simulink model "satPropWThrusterControlLinear"  (R2015b)
settings: Solver=ode45  StartTime=0.0  StopTime=tprop  RelTol=1e-8  AbsTol=1e-8
values from neighbouring files (symbols this model uses):
  epsilon0 = q(2:4)    [SetUp.m]
  eta0 = q(1)    [SetUp.m]
  J = [3500 0 0; 0 3200 0; 0 0 2500]    [SetUp.m]
  Jinv = inv(J)    [SetUp.m]
  kd = J*2*zeta*nf    [SetUp.m]
  kp = J*2*nf^2    [SetUp.m]
  mu = 398600    [COES2rvd.m]    (also in SetUp.m; test.m)
  n = 1/T    [SetUp.m]
  rvect = invconvmat*rvectx    [COES2rvd.m]    (also in test.m = rvect')
  vvect = invconvmat*vvectx    [COES2rvd.m]    (also in test.m = vvect')
  wbn0 = DCM*w    [SetUp.m]
settings Model: Creator=morganyost  LastModifiedBy=morganyost

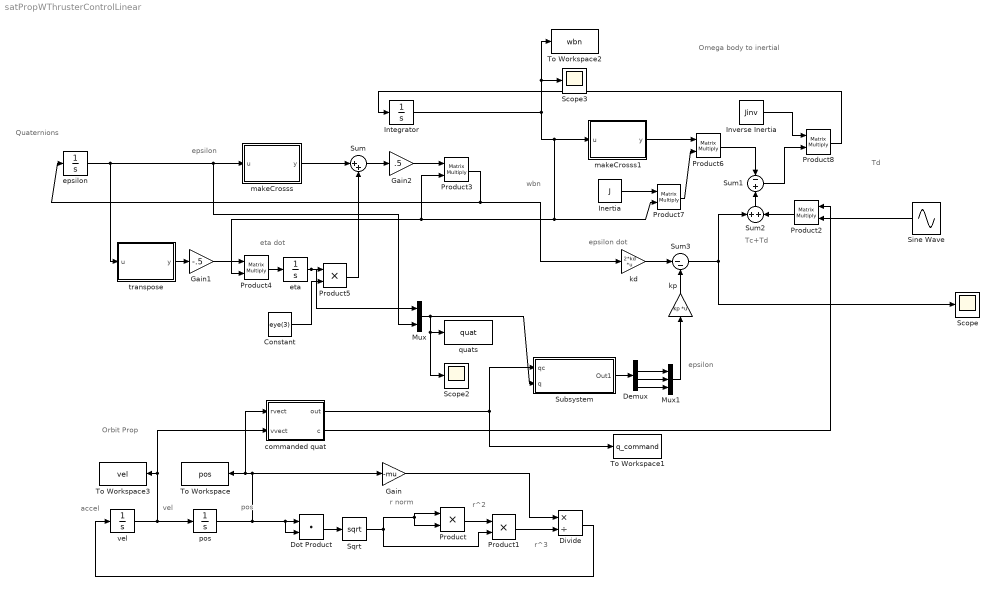
== system satPropWThrusterControlLinear ==
  note: epsilon
  note: epsilon dot
  note: Td
  note: Tc+Td
  note: Quaternions
  note: Omega body to inertial
  note: Orbit Prop
  note: eta dot
  note: wbn
  note: epsilon
  note: r^3
  note: r^2
  note: r norm
  note: pos
  note: vel
  note: accel
  Constant : Constant  Value=eye(3)
  Demux : Demux
  Divide : Product  Inputs=*/
  Dot Product : DotProduct  InputSameDT=on  OutDataTypeStr=Inherit: Inherit via internal rule
  Gain : Gain  Gain=-mu
  Gain1 : Gain  Gain=-.5
  Gain2 : Gain  Gain=.5
  Inertia : Constant  Value=J
  Integrator : Integrator  InitialCondition=wbn0
  Inverse Inertia : Constant  Value=Jinv
  Mux : Mux  Inputs=2
  Mux1 : Mux  Inputs=3
  Product : Product
  Product1 : Product
  Product{2..4,6..8} (6 alike) : Product  Multiplication=Matrix(*)
  Product5 : Product
  Scope : Scope
  Scope2 : Scope
  Scope3 : Scope
  Sine Wave : Sin  Amplitude=[0; 5e-7; 0]  Frequency=3*n  SampleTime=0
  Sqrt : Sqrt  SaturateOnIntegerOverflow=on
  Subsystem : Subsystem
  Sum : Sum  Inputs=|++
  Sum1 : Sum  Inputs=-+
  Sum2 : Sum
  Sum3 : Sum  Inputs=|--
  To Workspace : ToWorkspace  VariableName=pos  SaveFormat=Timeseries  SampleTime=-1
  To Workspace1 : ToWorkspace  VariableName=q_command  SaveFormat=Timeseries  SampleTime=-1
  To Workspace2 : ToWorkspace  VariableName=wbn  SaveFormat=Timeseries  SampleTime=-1
  To Workspace3 : ToWorkspace  VariableName=vel  SaveFormat=Timeseries  SampleTime=-1
  commanded quat : MATLAB Function  TreatAsAtomicUnit=on
  epsilon : Integrator  InitialCondition=epsilon0
  eta : Integrator  InitialCondition=eta0
  kd : Gain  Gain=2*kd  Multiplication=Matrix(K*u) (u vector)
  kp : Gain  Gain=kp  Multiplication=Matrix(K*u) (u vector)
  makeCrosss : MATLAB Function  TreatAsAtomicUnit=on
  makeCrosss1 : MATLAB Function  TreatAsAtomicUnit=on
  pos : Integrator  InitialCondition=rvect
  quats : ToWorkspace  VariableName=quat  SaveFormat=Timeseries  SampleTime=-1
  transpose : MATLAB Function  TreatAsAtomicUnit=on
  vel : Integrator  InitialCondition=vvect
  wires:
  vel/1 -> commanded quat/2(vvect), To Workspace3/1, pos/1
  pos/1 -> Gain/1, commanded quat/1(rvect), To Workspace/1, Dot Product/2, Dot Product/1
  Sqrt/1 -> Product/2, Product/1, Product1/2
  Product/1 -> Product1/1
  Product1/1 -> Divide/2
  Gain/1 -> Divide/1
  Divide/1 -> vel/1
  Dot Product/1 -> Sqrt/1
  epsilon/1 -> Mux/2, makeCrosss/1(u), transpose/1(u)
  makeCrosss/1(y) -> Sum/1
  eta/1 -> Mux/1, Product5/1
  Product5/1 -> Sum/2
  Sum/1 -> Gain2/1
  Gain2/1 -> Product3/1
  Product3/1 -> kd/1, epsilon/1
  Product4/1 -> eta/1
  transpose/1(y) -> Gain1/1
  Constant/1 -> Product5/2
  Gain1/1 -> Product4/1
  makeCrosss1/1(y) -> Product6/1
  Inertia/1 -> Product7/1
  Product7/1 -> Product6/2
  Inverse Inertia/1 -> Product8/1
  Product8/1 -> Integrator/1
  Mux/1 -> Subsystem/2(q), quats/1, Scope2/1
  Product6/1 -> Sum1/1
  Sum2/1 -> Sum1/2
  Sum3/1 -> Sum2/1, Scope/1
  kd/1 -> Sum3/1
  kp/1 -> Sum3/2
  Sum1/1 -> Product8/2
  Demux/4 -> Mux1/3
  Demux/3 -> Mux1/2
  Demux/2 -> Mux1/1
  Mux1/1 -> kp/1
  Subsystem/1(Out1) -> Demux/1
  commanded quat/1(out) -> To Workspace1/1, Subsystem/1(qc)
  commanded quat/2(c) -> Product2/1
  Sine Wave/1 -> Product2/2
  Product2/1 -> Sum2/2
  Integrator/1 -> Product7/2, Product3/2, Product4/2, makeCrosss1/1(u), To Workspace2/1, Scope3/1

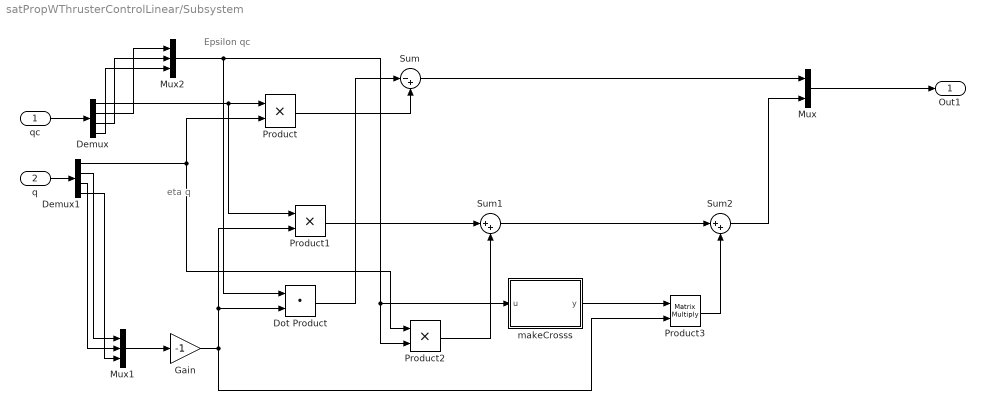
== system satPropWThrusterControlLinear/Subsystem ==
  note: eta q
  note: Epsilon qc
  qc : Inport
  q : Inport  Port=2
  Demux : Demux
  Demux1 : Demux
  Dot Product : DotProduct  InputSameDT=on  OutDataTypeStr=Inherit: Inherit via internal rule
  Gain : Gain  Gain=-1
  Mux : Mux  Inputs=2
  Mux1 : Mux  Inputs=3
  Mux2 : Mux  Inputs=3
  Product : Product
  Product1 : Product
  Product2 : Product
  Product3 : Product  Multiplication=Matrix(*)
  Sum : Sum  Inputs=|-+
  Sum1 : Sum  Inputs=|++
  Sum2 : Sum  Inputs=|++
  makeCrosss : MATLAB Function  TreatAsAtomicUnit=on
  Out1 : Outport
  wires:
  qc/1 -> Demux/1
  q/1 -> Demux1/1
  Demux/1 -> Product1/1, Product/1
  Demux1/1 -> Product2/1, Product/2
  Product/1 -> Sum/2
  Demux/2 -> Mux2/1
  Demux/3 -> Mux2/2
  Demux/4 -> Mux2/3
  Demux1/2 -> Mux1/1
  Demux1/3 -> Mux1/2
  Demux1/4 -> Mux1/3
  Mux2/1 -> Product2/2, makeCrosss/1(u), Dot Product/1
  Mux1/1 -> Gain/1
  Dot Product/1 -> Sum/1
  Sum/1 -> Mux/1
  Product1/1 -> Sum1/1
  Product2/1 -> Sum1/2
  Sum1/1 -> Sum2/1
  Product3/1 -> Sum2/2
  makeCrosss/1(y) -> Product3/1
  Gain/1 -> Product1/2, Dot Product/2, Product3/2
  Sum2/1 -> Mux/2
  Mux/1 -> Out1/1

== matlab function satPropWThrusterControlLinear/makeCrosss ==
  data: u input; y output
function y = fcn(u)
%#codegen
Ex = u(1);
Ey = u(2);
Ez = u(3);

y = [0 -Ez Ey; Ez 0 -Ex; -Ey Ex 0];

== matlab function satPropWThrusterControlLinear/Subsystem/makeCrosss ==
  data: u input; y output
function y = fcn(u)
%#codegen
Ex = u(1);
Ey = u(2);
Ez = u(3);

y = [0 -Ez Ey; Ez 0 -Ex; -Ey Ex 0];

== matlab function satPropWThrusterControlLinear/transpose ==
  data: u input; y output
function y = fcn(u)
%#codegen

y = u';

== matlab function satPropWThrusterControlLinear/makeCrosss1 ==
  data: u input; y output
function y = fcn(u)
%#codegen
Ex = u(1);
Ey = u(2);
Ez = u(3);

y = [0 -Ez Ey; Ez 0 -Ex; -Ey Ex 0];

== matlab function satPropWThrusterControlLinear/commanded quat ==
  data: rvect input; out output; vvect input; c output
function [out, c]= fcn(rvect, vvect)
%#codegen
h_a = cross(rvect,vvect);
k_hat = -rvect/norm(rvect);
j_hat = -h_a/norm(h_a);
i_hat = cross(j_hat, k_hat);
x = [1 0 0];
y = [0 1 0];
z = [0 0 1];
c = [dot(x, i_hat) dot(x, j_hat) dot(x, k_hat);
       dot(y, i_hat) dot(y, j_hat) dot(y, k_hat);
       dot(z, i_hat) dot(z, j_hat) dot(z, k_hat)];
out = DCM2quat(c);
